simulink model "building_PHPP_v1"  (R2018b)
settings: Solver=ode23s  StartTime=-building.preruntime+8760*3600  StopTime=building.runtime+8760*3600  EnableMultiTasking=on
StartFcn:
  | tic
StopFcn:
  | toc
values from neighbouring files (symbols this model uses):
  A = 7*10*2    (= 140)    [theta_ground_v1.m]    (also in xlswrite1.m = num2cell(data))
  B = A/(0.5 * P)    (= 8.23529411765)    [theta_ground_v1.m]
  building = obj    [BUILDING.m]    (also in create_building_automatic.m = building.save(); ini_building_automatic.m = building.add_variant_hvac(building.variant_hvac, hvac); load_building_automatic.m = building.save())
  C = zeros(1,length(d)+1)    [CONSTRUCTION.m]    (also in DOOR.m = [0 0 0]; WALL.m = [0 0 0]; WINDOW.m = [0 0 0])
  cp = str2num(value)    [CONSTRUCTION.m]
  p = [timevec_weather weather(:,12)]    [BOUNDARY.m]    (also in WEATHER.m = 0; init_carnotUIBK.m = cell2mat(carnotUIBKpaths(i,2)))
  rho = str2num(value)    [CONSTRUCTION.m]    (also in theta_ground_v1.m = 2000)
undefined symbols (not defined in the file or in its folder): Dd, Dreifach, get_building, Qdot_C, Qdot_C_energy, Qdot_H, Qdot_H_energy, Qdot_I_electricity, Qdot_I_electricity_energy, Qdot_I_light, Qdot_I_light_energy, Qdot_I_person, Qdot_I_person_energy, Qdot_S, Qdot_S_energy, Qdot_T_ground, Qdot_T_ground_energy, Qdot_T_neighbour, Qdot_T_neighbour_energy, Qdot_T_opaque, Qdot_T_opaque_energy, Qdot_T_window, Qdot_T_window_energy, Qdot_V_infiltration, Qdot_V_infiltration_energy, Qdot_V_mech, Qdot_V_mech_energy, Qdot_V_window, Qdot_V_window_energy, Tc, Tr, Ts, Wärmeschutzglas, x_CO2, x_H2O, x_VOC
libraries: carnotUIBK x1874, carnot x5, simulink x3
(part 32 of 34)

== system building_PHPP_v1/BUILDING/ZONE_9/gain_4 ==
  AIB : Inport
  control : Inport  Port=2
  EMPTY : carnotUIBK/gain/EMPTY  SystemSampleTime=-1  VariantControl=(default)
  Equipment : carnotUIBK/gain/Equipment  SystemSampleTime=-1  VariantControl=V_z9_i4_m2
  Light : carnotUIBK/gain/Light  SystemSampleTime=-1  VariantControl=V_z9_i4_m1
  Moisture : carnotUIBK/gain/Moisture  SystemSampleTime=-1  VariantControl=V_z9_i4_m3
  People : carnotUIBK/gain/People  SystemSampleTime=-1  VariantControl=V_z9_i4_m0
  "[S]" : Outport

== system building_PHPP_v1/BUILDING/ZONE_9/gain_5 ==
  AIB : Inport
  control : Inport  Port=2
  EMPTY : carnotUIBK/gain/EMPTY  SystemSampleTime=-1  VariantControl=(default)
  Equipment : carnotUIBK/gain/Equipment  SystemSampleTime=-1  VariantControl=V_z9_i5_m2
  Light : carnotUIBK/gain/Light  SystemSampleTime=-1  VariantControl=V_z9_i5_m1
  Moisture : carnotUIBK/gain/Moisture  SystemSampleTime=-1  VariantControl=V_z9_i5_m3
  People : carnotUIBK/gain/People  SystemSampleTime=-1  VariantControl=V_z9_i5_m0
  "[S]" : Outport

== system building_PHPP_v1/BUILDING/ZONE_9/infiltration_1 ==
  AIB : Inport
  WDB : Inport  Port=2
  control : Inport  Port=3
  EMPTY : carnotUIBK/infiltration/EMPTY  VariantControl=(default)
  infiltration_constant : carnotUIBK/infiltration/infiltration_constant  VariantControl=V_z9_inf1_m0  volume=z.heated_volume  n50=z.n50  wind_e=0.07  co2=400
  infiltration_pressure : carnotUIBK/infiltration/infiltration_pressure  VariantControl=V_z9_inf1_m1  volume=z.heated_volume  n50=z.n50  wind_e=0.07  co2=400
  "[S]" : Outport

== system building_PHPP_v1/BUILDING/ZONE_9/infiltration_2 ==
  AIB : Inport
  WDB : Inport  Port=2
  control : Inport  Port=3
  EMPTY : carnotUIBK/infiltration/EMPTY  VariantControl=(default)
  infiltration_constant : carnotUIBK/infiltration/infiltration_constant  VariantControl=V_z9_inf2_m0  volume=z.heated_volume  n50=z.n50  wind_e=0.07  co2=400
  infiltration_pressure : carnotUIBK/infiltration/infiltration_pressure  VariantControl=V_z9_inf2_m1  volume=z.heated_volume  n50=z.n50  wind_e=0.07  co2=400
  "[S]" : Outport

== system building_PHPP_v1/BUILDING/ZONE_9/infiltration_3 ==
  AIB : Inport
  WDB : Inport  Port=2
  control : Inport  Port=3
  EMPTY : carnotUIBK/infiltration/EMPTY  VariantControl=(default)
  infiltration_constant : carnotUIBK/infiltration/infiltration_constant  VariantControl=V_z9_inf3_m0  volume=z.heated_volume  n50=z.n50  wind_e=0.07  co2=400
  infiltration_pressure : carnotUIBK/infiltration/infiltration_pressure  VariantControl=V_z9_inf3_m1  volume=z.heated_volume  n50=z.n50  wind_e=0.07  co2=400
  "[S]" : Outport

== system building_PHPP_v1/BUILDING/ZONE_9/infiltration_4 ==
  AIB : Inport
  WDB : Inport  Port=2
  control : Inport  Port=3
  EMPTY : carnotUIBK/infiltration/EMPTY  VariantControl=(default)
  infiltration_constant : carnotUIBK/infiltration/infiltration_constant  VariantControl=V_z9_inf4_m0  volume=z.heated_volume  n50=z.n50  wind_e=0.07  co2=400
  infiltration_pressure : carnotUIBK/infiltration/infiltration_pressure  VariantControl=V_z9_inf4_m1  volume=z.heated_volume  n50=z.n50  wind_e=0.07  co2=400
  "[S]" : Outport

== system building_PHPP_v1/BUILDING/ZONE_9/infiltration_5 ==
  AIB : Inport
  WDB : Inport  Port=2
  control : Inport  Port=3
  EMPTY : carnotUIBK/infiltration/EMPTY  VariantControl=(default)
  infiltration_constant : carnotUIBK/infiltration/infiltration_constant  VariantControl=V_z9_inf5_m0  volume=z.heated_volume  n50=z.n50  wind_e=0.07  co2=400
  infiltration_pressure : carnotUIBK/infiltration/infiltration_pressure  VariantControl=V_z9_inf5_m1  volume=z.heated_volume  n50=z.n50  wind_e=0.07  co2=400
  "[S]" : Outport

== system building_PHPP_v1/BUILDING/ZONE_9/room_node ==
  sum([S]) : Inport
  1-node : carnotUIBK/room_node/1-node  VariantControl=V_z9_m2  zoneairvolume=z.heated_volume  zoneheight=z.heated_volume/z.heated_area  zonestartTEMP=z.t_ini  zonestartWATER=z.phi_ini  zonestartCO2=z.CO2_ini  zonestartVOC=z.VOC_ini  zonestartP0=1e5/(293.15)*(273.15+z.t_ini)  timeconst=z.timeconstant  mcp=z.cp_spec*z.heated_area
  1-node_womass : carnotUIBK/room_node/1-node_womass  VariantControl=V_z9_m4  zoneairvolume=z.heated_volume  zoneheight=z.heated_volume/z.heated_area  zonestartTEMP=z.t_ini  zonestartWATER=z.phi_ini  zonestartCO2=z.CO2_ini  zonestartVOC=z.VOC_ini  zonestartP0=1e5/(293.15)*(273.15+z.t_ini)  timeconst=z.timeconstant  mcp=z.cp_spec*z.heated_area
  2-node : carnotUIBK/room_node/2-node  VariantControl=V_z9_m3  zoneairvolume=z.heated_volume  zoneheight=z.heated_volume/z.heated_area  zonestartTEMP=z.t_ini  zonestartWATER=z.phi_ini  zonestartCO2=z.CO2_ini  zonestartVOC=z.VOC_ini  zonestartP0=1e5/(293.15)*(273.15+z.t_ini)  timeconst=z.timeconstant
  2-node_ideal : carnotUIBK/room_node/2-node_ideal  VariantControl=V_z9_m1  zoneairvolume=z.heated_volume  zoneheight=z.heated_volume/z.heated_area  zonestartTEMP=z.t_ini  zonestartWATER=z.phi_ini  zonestartCO2=z.CO2_ini  zonestartVOC=z.VOC_ini  zonestartP0=1e5/(293.15)*(273.15+z.t_ini)  timeconst=z.timeconstant  temperature_timevalues=z.profile_timevalues  temperature_timeduration=z.profile_timeduration  temperature_Tc=z.profile_Tc  temperature_Tr=z.profile_Tc
  EMPTY : carnotUIBK/room_node/EMPTY  VariantControl=(default)  temperature_timevalues=z.profile_timevalues  temperature_timeduration=z.profile_timeduration  temperature_Tc=z.profile_Tc  temperature_Tr=z.profile_Tr  temperature_rH=z.profile_rH  temperature_CO2=z.profile_CO2  temperature_VOC=z.profile_VOC  temperature_p=z.profile_p
  BDB : Outport
  AIB : Outport  Port=2
  Qdot_sol : Outport  Port=3

== system building_PHPP_v1/BUILDING/ZONE_9/wall_1 ==
  WDB : Inport
  GDB : Inport  Port=2
  NDB : Inport  Port=3
  AIB : Inport  Port=4
  Qdot_in : Inport  Port=5
  Qdot_sol : Inport  Port=6
  EMPTY : carnotUIBK/wall_zone/EMPTY  VariantControl=(default)
  R-C model : carnotUIBK/wall_zone/R-C model  VariantControl=V_z9_w1_m1  t0=z.t_ini  d=fliplr(const.parameter.xmesh_beu)  cond=fliplr(const.parameter.lambda)  cwall=fliplr(const.parameter.cp)  rho=fliplr(const.parameter.rho)  reflectground=0.2  abs_emiss=[const.absorption_2 const.emission_2 const.emission_1]  tau=const.parameter.tau  dactive=const.parameter.d_active
      link override alpha_e/alpha_e_AMBIENT: VariantControl=V_z9_w1_hte0
      link override alpha_e/alpha_e_GROUND: VariantControl=V_z9_w1_hte1
      link override alpha_e/alpha_e_INTERNAL: VariantControl=V_z9_w1_hte2
      link override alpha_e/alpha_e_INTERNAL/alpha_i/alpha_i_down: VariantControl=V_z9_w1_hti2
      link override alpha_e/alpha_e_INTERNAL/alpha_i/alpha_i_horizontal: VariantControl=V_z9_w1_hti0
      link override alpha_e/alpha_e_INTERNAL/alpha_i/alpha_i_up: VariantControl=V_z9_w1_hti1
      link override alpha_e/alpha_e_NEIGHBOUR: VariantControl=V_z9_w1_hte3
      link override alpha_e/alpha_e_NEIGHBOUR/alpha_i/alpha_i_down: VariantControl=V_z9_w1_hti2
      link override alpha_e/alpha_e_NEIGHBOUR/alpha_i/alpha_i_horizontal: VariantControl=V_z9_w1_hti0
      link override alpha_e/alpha_e_NEIGHBOUR/alpha_i/alpha_i_up: VariantControl=V_z9_w1_hti1
      link override alpha_i/alpha_i_down: VariantControl=V_z9_w1_hti2
      link override alpha_i/alpha_i_horizontal: VariantControl=V_z9_w1_hti0
      link override alpha_i/alpha_i_up: VariantControl=V_z9_w1_hti1
  UA : carnotUIBK/wall_zone/UA  VariantControl=V_z9_w1_m0  U=const.parameter.U
      link override Rse/AMBIENT: VariantControl=V_z9_w1_hte0
      link override Rse/GROUND: VariantControl=V_z9_w1_hte1
      link override Rse/INTERNAL: VariantControl=V_z9_w1_hte2
      link override Rse/NEIGHBOUR: VariantControl=V_z9_w1_hte3
      link override Rsi/down: VariantControl=V_z9_w1_hti2
      link override Rsi/horizontal: VariantControl=V_z9_w1_hti0
      link override Rsi/up: VariantControl=V_z9_w1_hti1
  hygrothermal model : carnotUIBK/wall_zone/hygrothermal model  VariantControl=V_z9_w1_m2  t0=z.t_ini  reflectground=0.2  abs_emiss=[const.absorption_2 const.emission_2 const.emission_1]  xmesh=const.parameter.xmesh_hygro  X=const.parameter.X  d=const.parameter.d  lambda=const.parameter.lambda_hygro  rho=const.parameter.rho_hygro  cp=const.parameter.cp_hygro  mu=const.parameter.mu  ufs=const.parameter.ufs  FSF_u=const.parameter.FSF_u  FSF_phi=const.parameter.FSF_phi  FSF_dudphi=const.parameter.FSF_dudphi  FSF_k=const.parameter.FSF_k  K_kleff=const.parameter.K_kleff  K_u=const.parameter.K_u  K_kl=const.parameter.K_kl  FSF_length=const.parameter.FSF_length  K_length=const.parameter.K_length  T_ini=const.parameter.T_ini_hygro  Phi_ini=const.parameter.Phi_ini_hygro  T_source=const.parameter.T_source  Phi_source=const.parameter.Phi_source  Tdactive=const.parameter.T_dactive  Phidactive=const.parameter.Phi_dactive
      link override alpha_e/alpha_e_AMBIENT: VariantControl=V_z9_w1_hte0
      link override alpha_e/alpha_e_GROUND: VariantControl=V_z9_w1_hte1
      link override alpha_e/alpha_e_INTERNAL: VariantControl=V_z9_w1_hte2
      link override alpha_e/alpha_e_INTERNAL/alpha_i/alpha_i_down: VariantControl=V_z9_w1_hti2
      link override alpha_e/alpha_e_INTERNAL/alpha_i/alpha_i_horizontal: VariantControl=V_z9_w1_hti0
      link override alpha_e/alpha_e_INTERNAL/alpha_i/alpha_i_up: VariantControl=V_z9_w1_hti1
      link override alpha_e/alpha_e_NEIGHBOUR: VariantControl=V_z9_w1_hte3
      link override alpha_e/alpha_e_NEIGHBOUR/alpha_i/alpha_i_down: VariantControl=V_z9_w1_hti2
      link override alpha_e/alpha_e_NEIGHBOUR/alpha_i/alpha_i_horizontal: VariantControl=V_z9_w1_hti0
      link override alpha_e/alpha_e_NEIGHBOUR/alpha_i/alpha_i_up: VariantControl=V_z9_w1_hti1
      link override alpha_i/alpha_i_down: VariantControl=V_z9_w1_hti2
      link override alpha_i/alpha_i_horizontal: VariantControl=V_z9_w1_hti0
      link override alpha_i/alpha_i_up: VariantControl=V_z9_w1_hti1
  "[S]" : Outport
  theta_out : Outport  Port=2

== system building_PHPP_v1/BUILDING/ZONE_9/wall_2 ==
  WDB : Inport
  GDB : Inport  Port=2
  NDB : Inport  Port=3
  AIB : Inport  Port=4
  Qdot_in : Inport  Port=5
  Qdot_sol : Inport  Port=6
  EMPTY : carnotUIBK/wall_zone/EMPTY  VariantControl=(default)
  R-C model : carnotUIBK/wall_zone/R-C model  VariantControl=V_z9_w2_m1  t0=z.t_ini  d=fliplr(const.parameter.xmesh_beu)  cond=fliplr(const.parameter.lambda)  cwall=fliplr(const.parameter.cp)  rho=fliplr(const.parameter.rho)  reflectground=0.2  abs_emiss=[const.absorption_2 const.emission_2 const.emission_1]  tau=const.parameter.tau  dactive=const.parameter.d_active
      link override alpha_e/alpha_e_AMBIENT: VariantControl=V_z9_w2_hte0
      link override alpha_e/alpha_e_GROUND: VariantControl=V_z9_w2_hte1
      link override alpha_e/alpha_e_INTERNAL: VariantControl=V_z9_w2_hte2
      link override alpha_e/alpha_e_INTERNAL/alpha_i/alpha_i_down: VariantControl=V_z9_w2_hti2
      link override alpha_e/alpha_e_INTERNAL/alpha_i/alpha_i_horizontal: VariantControl=V_z9_w2_hti0
      link override alpha_e/alpha_e_INTERNAL/alpha_i/alpha_i_up: VariantControl=V_z9_w2_hti1
      link override alpha_e/alpha_e_NEIGHBOUR: VariantControl=V_z9_w2_hte3
      link override alpha_e/alpha_e_NEIGHBOUR/alpha_i/alpha_i_down: VariantControl=V_z9_w2_hti2
      link override alpha_e/alpha_e_NEIGHBOUR/alpha_i/alpha_i_horizontal: VariantControl=V_z9_w2_hti0
      link override alpha_e/alpha_e_NEIGHBOUR/alpha_i/alpha_i_up: VariantControl=V_z9_w2_hti1
      link override alpha_i/alpha_i_down: VariantControl=V_z9_w2_hti2
      link override alpha_i/alpha_i_horizontal: VariantControl=V_z9_w2_hti0
      link override alpha_i/alpha_i_up: VariantControl=V_z9_w2_hti1
  UA : carnotUIBK/wall_zone/UA  VariantControl=V_z9_w2_m0  U=const.parameter.U
      link override Rse/AMBIENT: VariantControl=V_z9_w2_hte0
      link override Rse/GROUND: VariantControl=V_z9_w2_hte1
      link override Rse/INTERNAL: VariantControl=V_z9_w2_hte2
      link override Rse/NEIGHBOUR: VariantControl=V_z9_w2_hte3
      link override Rsi/down: VariantControl=V_z9_w2_hti2
      link override Rsi/horizontal: VariantControl=V_z9_w2_hti0
      link override Rsi/up: VariantControl=V_z9_w2_hti1
  hygrothermal model : carnotUIBK/wall_zone/hygrothermal model  VariantControl=V_z9_w2_m2  t0=z.t_ini  reflectground=0.2  abs_emiss=[const.absorption_2 const.emission_2 const.emission_1]  xmesh=const.parameter.xmesh_hygro  X=const.parameter.X  d=const.parameter.d  lambda=const.parameter.lambda_hygro  rho=const.parameter.rho_hygro  cp=const.parameter.cp_hygro  mu=const.parameter.mu  ufs=const.parameter.ufs  FSF_u=const.parameter.FSF_u  FSF_phi=const.parameter.FSF_phi  FSF_dudphi=const.parameter.FSF_dudphi  FSF_k=const.parameter.FSF_k  K_kleff=const.parameter.K_kleff  K_u=const.parameter.K_u  K_kl=const.parameter.K_kl  FSF_length=const.parameter.FSF_length  K_length=const.parameter.K_length  T_ini=const.parameter.T_ini_hygro  Phi_ini=const.parameter.Phi_ini_hygro  T_source=const.parameter.T_source  Phi_source=const.parameter.Phi_source  Tdactive=const.parameter.T_dactive  Phidactive=const.parameter.Phi_dactive
      link override alpha_e/alpha_e_AMBIENT: VariantControl=V_z9_w2_hte0
      link override alpha_e/alpha_e_GROUND: VariantControl=V_z9_w2_hte1
      link override alpha_e/alpha_e_INTERNAL: VariantControl=V_z9_w2_hte2
      link override alpha_e/alpha_e_INTERNAL/alpha_i/alpha_i_down: VariantControl=V_z9_w2_hti2
      link override alpha_e/alpha_e_INTERNAL/alpha_i/alpha_i_horizontal: VariantControl=V_z9_w2_hti0
      link override alpha_e/alpha_e_INTERNAL/alpha_i/alpha_i_up: VariantControl=V_z9_w2_hti1
      link override alpha_e/alpha_e_NEIGHBOUR: VariantControl=V_z9_w2_hte3
      link override alpha_e/alpha_e_NEIGHBOUR/alpha_i/alpha_i_down: VariantControl=V_z9_w2_hti2
      link override alpha_e/alpha_e_NEIGHBOUR/alpha_i/alpha_i_horizontal: VariantControl=V_z9_w2_hti0
      link override alpha_e/alpha_e_NEIGHBOUR/alpha_i/alpha_i_up: VariantControl=V_z9_w2_hti1
      link override alpha_i/alpha_i_down: VariantControl=V_z9_w2_hti2
      link override alpha_i/alpha_i_horizontal: VariantControl=V_z9_w2_hti0
      link override alpha_i/alpha_i_up: VariantControl=V_z9_w2_hti1
  "[S]" : Outport
  theta_out : Outport  Port=2

== system building_PHPP_v1/BUILDING/ZONE_9/wall_3 ==
  WDB : Inport
  GDB : Inport  Port=2
  NDB : Inport  Port=3
  AIB : Inport  Port=4
  Qdot_in : Inport  Port=5
  Qdot_sol : Inport  Port=6
  EMPTY : carnotUIBK/wall_zone/EMPTY  VariantControl=(default)
  R-C model : carnotUIBK/wall_zone/R-C model  VariantControl=V_z9_w3_m1  t0=z.t_ini  d=fliplr(const.parameter.xmesh_beu)  cond=fliplr(const.parameter.lambda)  cwall=fliplr(const.parameter.cp)  rho=fliplr(const.parameter.rho)  reflectground=0.2  abs_emiss=[const.absorption_2 const.emission_2 const.emission_1]  tau=const.parameter.tau  dactive=const.parameter.d_active
      link override alpha_e/alpha_e_AMBIENT: VariantControl=V_z9_w3_hte0
      link override alpha_e/alpha_e_GROUND: VariantControl=V_z9_w3_hte1
      link override alpha_e/alpha_e_INTERNAL: VariantControl=V_z9_w3_hte2
      link override alpha_e/alpha_e_INTERNAL/alpha_i/alpha_i_down: VariantControl=V_z9_w3_hti2
      link override alpha_e/alpha_e_INTERNAL/alpha_i/alpha_i_horizontal: VariantControl=V_z9_w3_hti0
      link override alpha_e/alpha_e_INTERNAL/alpha_i/alpha_i_up: VariantControl=V_z9_w3_hti1
      link override alpha_e/alpha_e_NEIGHBOUR: VariantControl=V_z9_w3_hte3
      link override alpha_e/alpha_e_NEIGHBOUR/alpha_i/alpha_i_down: VariantControl=V_z9_w3_hti2
      link override alpha_e/alpha_e_NEIGHBOUR/alpha_i/alpha_i_horizontal: VariantControl=V_z9_w3_hti0
      link override alpha_e/alpha_e_NEIGHBOUR/alpha_i/alpha_i_up: VariantControl=V_z9_w3_hti1
      link override alpha_i/alpha_i_down: VariantControl=V_z9_w3_hti2
      link override alpha_i/alpha_i_horizontal: VariantControl=V_z9_w3_hti0
      link override alpha_i/alpha_i_up: VariantControl=V_z9_w3_hti1
  UA : carnotUIBK/wall_zone/UA  VariantControl=V_z9_w3_m0  U=const.parameter.U
      link override Rse/AMBIENT: VariantControl=V_z9_w3_hte0
      link override Rse/GROUND: VariantControl=V_z9_w3_hte1
      link override Rse/INTERNAL: VariantControl=V_z9_w3_hte2
      link override Rse/NEIGHBOUR: VariantControl=V_z9_w3_hte3
      link override Rsi/down: VariantControl=V_z9_w3_hti2
      link override Rsi/horizontal: VariantControl=V_z9_w3_hti0
      link override Rsi/up: VariantControl=V_z9_w3_hti1
  hygrothermal model : carnotUIBK/wall_zone/hygrothermal model  VariantControl=V_z9_w3_m2  t0=z.t_ini  reflectground=0.2  abs_emiss=[const.absorption_2 const.emission_2 const.emission_1]  xmesh=const.parameter.xmesh_hygro  X=const.parameter.X  d=const.parameter.d  lambda=const.parameter.lambda_hygro  rho=const.parameter.rho_hygro  cp=const.parameter.cp_hygro  mu=const.parameter.mu  ufs=const.parameter.ufs  FSF_u=const.parameter.FSF_u  FSF_phi=const.parameter.FSF_phi  FSF_dudphi=const.parameter.FSF_dudphi  FSF_k=const.parameter.FSF_k  K_kleff=const.parameter.K_kleff  K_u=const.parameter.K_u  K_kl=const.parameter.K_kl  FSF_length=const.parameter.FSF_length  K_length=const.parameter.K_length  T_ini=const.parameter.T_ini_hygro  Phi_ini=const.parameter.Phi_ini_hygro  T_source=const.parameter.T_source  Phi_source=const.parameter.Phi_source  Tdactive=const.parameter.T_dactive  Phidactive=const.parameter.Phi_dactive
      link override alpha_e/alpha_e_AMBIENT: VariantControl=V_z9_w3_hte0
      link override alpha_e/alpha_e_GROUND: VariantControl=V_z9_w3_hte1
      link override alpha_e/alpha_e_INTERNAL: VariantControl=V_z9_w3_hte2
      link override alpha_e/alpha_e_INTERNAL/alpha_i/alpha_i_down: VariantControl=V_z9_w3_hti2
      link override alpha_e/alpha_e_INTERNAL/alpha_i/alpha_i_horizontal: VariantControl=V_z9_w3_hti0
      link override alpha_e/alpha_e_INTERNAL/alpha_i/alpha_i_up: VariantControl=V_z9_w3_hti1
      link override alpha_e/alpha_e_NEIGHBOUR: VariantControl=V_z9_w3_hte3
      link override alpha_e/alpha_e_NEIGHBOUR/alpha_i/alpha_i_down: VariantControl=V_z9_w3_hti2
      link override alpha_e/alpha_e_NEIGHBOUR/alpha_i/alpha_i_horizontal: VariantControl=V_z9_w3_hti0
      link override alpha_e/alpha_e_NEIGHBOUR/alpha_i/alpha_i_up: VariantControl=V_z9_w3_hti1
      link override alpha_i/alpha_i_down: VariantControl=V_z9_w3_hti2
      link override alpha_i/alpha_i_horizontal: VariantControl=V_z9_w3_hti0
      link override alpha_i/alpha_i_up: VariantControl=V_z9_w3_hti1
  "[S]" : Outport
  theta_out : Outport  Port=2

== system building_PHPP_v1/BUILDING/ZONE_9/wall_4 ==
  WDB : Inport
  GDB : Inport  Port=2
  NDB : Inport  Port=3
  AIB : Inport  Port=4
  Qdot_in : Inport  Port=5
  Qdot_sol : Inport  Port=6
  EMPTY : carnotUIBK/wall_zone/EMPTY  VariantControl=(default)
  R-C model : carnotUIBK/wall_zone/R-C model  VariantControl=V_z9_w4_m1  t0=z.t_ini  d=fliplr(const.parameter.xmesh_beu)  cond=fliplr(const.parameter.lambda)  cwall=fliplr(const.parameter.cp)  rho=fliplr(const.parameter.rho)  reflectground=0.2  abs_emiss=[const.absorption_2 const.emission_2 const.emission_1]  tau=const.parameter.tau  dactive=const.parameter.d_active
      link override alpha_e/alpha_e_AMBIENT: VariantControl=V_z9_w4_hte0
      link override alpha_e/alpha_e_GROUND: VariantControl=V_z9_w4_hte1
      link override alpha_e/alpha_e_INTERNAL: VariantControl=V_z9_w4_hte2
      link override alpha_e/alpha_e_INTERNAL/alpha_i/alpha_i_down: VariantControl=V_z9_w4_hti2
      link override alpha_e/alpha_e_INTERNAL/alpha_i/alpha_i_horizontal: VariantControl=V_z9_w4_hti0
      link override alpha_e/alpha_e_INTERNAL/alpha_i/alpha_i_up: VariantControl=V_z9_w4_hti1
      link override alpha_e/alpha_e_NEIGHBOUR: VariantControl=V_z9_w4_hte3
      link override alpha_e/alpha_e_NEIGHBOUR/alpha_i/alpha_i_down: VariantControl=V_z9_w4_hti2
      link override alpha_e/alpha_e_NEIGHBOUR/alpha_i/alpha_i_horizontal: VariantControl=V_z9_w4_hti0
      link override alpha_e/alpha_e_NEIGHBOUR/alpha_i/alpha_i_up: VariantControl=V_z9_w4_hti1
      link override alpha_i/alpha_i_down: VariantControl=V_z9_w4_hti2
      link override alpha_i/alpha_i_horizontal: VariantControl=V_z9_w4_hti0
      link override alpha_i/alpha_i_up: VariantControl=V_z9_w4_hti1
  UA : carnotUIBK/wall_zone/UA  VariantControl=V_z9_w4_m0  U=const.parameter.U
      link override Rse/AMBIENT: VariantControl=V_z9_w4_hte0
      link override Rse/GROUND: VariantControl=V_z9_w4_hte1
      link override Rse/INTERNAL: VariantControl=V_z9_w4_hte2
      link override Rse/NEIGHBOUR: VariantControl=V_z9_w4_hte3
      link override Rsi/down: VariantControl=V_z9_w4_hti2
      link override Rsi/horizontal: VariantControl=V_z9_w4_hti0
      link override Rsi/up: VariantControl=V_z9_w4_hti1
  hygrothermal model : carnotUIBK/wall_zone/hygrothermal model  VariantControl=V_z9_w4_m2  t0=z.t_ini  reflectground=0.2  abs_emiss=[const.absorption_2 const.emission_2 const.emission_1]  xmesh=const.parameter.xmesh_hygro  X=const.parameter.X  d=const.parameter.d  lambda=const.parameter.lambda_hygro  rho=const.parameter.rho_hygro  cp=const.parameter.cp_hygro  mu=const.parameter.mu  ufs=const.parameter.ufs  FSF_u=const.parameter.FSF_u  FSF_phi=const.parameter.FSF_phi  FSF_dudphi=const.parameter.FSF_dudphi  FSF_k=const.parameter.FSF_k  K_kleff=const.parameter.K_kleff  K_u=const.parameter.K_u  K_kl=const.parameter.K_kl  FSF_length=const.parameter.FSF_length  K_length=const.parameter.K_length  T_ini=const.parameter.T_ini_hygro  Phi_ini=const.parameter.Phi_ini_hygro  T_source=const.parameter.T_source  Phi_source=const.parameter.Phi_source  Tdactive=const.parameter.T_dactive  Phidactive=const.parameter.Phi_dactive
      link override alpha_e/alpha_e_AMBIENT: VariantControl=V_z9_w4_hte0
      link override alpha_e/alpha_e_GROUND: VariantControl=V_z9_w4_hte1
      link override alpha_e/alpha_e_INTERNAL: VariantControl=V_z9_w4_hte2
      link override alpha_e/alpha_e_INTERNAL/alpha_i/alpha_i_down: VariantControl=V_z9_w4_hti2
      link override alpha_e/alpha_e_INTERNAL/alpha_i/alpha_i_horizontal: VariantControl=V_z9_w4_hti0
      link override alpha_e/alpha_e_INTERNAL/alpha_i/alpha_i_up: VariantControl=V_z9_w4_hti1
      link override alpha_e/alpha_e_NEIGHBOUR: VariantControl=V_z9_w4_hte3
      link override alpha_e/alpha_e_NEIGHBOUR/alpha_i/alpha_i_down: VariantControl=V_z9_w4_hti2
      link override alpha_e/alpha_e_NEIGHBOUR/alpha_i/alpha_i_horizontal: VariantControl=V_z9_w4_hti0
      link override alpha_e/alpha_e_NEIGHBOUR/alpha_i/alpha_i_up: VariantControl=V_z9_w4_hti1
      link override alpha_i/alpha_i_down: VariantControl=V_z9_w4_hti2
      link override alpha_i/alpha_i_horizontal: VariantControl=V_z9_w4_hti0
      link override alpha_i/alpha_i_up: VariantControl=V_z9_w4_hti1
  "[S]" : Outport
  theta_out : Outport  Port=2

== system building_PHPP_v1/BUILDING/ZONE_9/wall_5 ==
  WDB : Inport
  GDB : Inport  Port=2
  NDB : Inport  Port=3
  AIB : Inport  Port=4
  Qdot_in : Inport  Port=5
  Qdot_sol : Inport  Port=6
  EMPTY : carnotUIBK/wall_zone/EMPTY  VariantControl=(default)
  R-C model : carnotUIBK/wall_zone/R-C model  VariantControl=V_z9_w5_m1  t0=z.t_ini  d=fliplr(const.parameter.xmesh_beu)  cond=fliplr(const.parameter.lambda)  cwall=fliplr(const.parameter.cp)  rho=fliplr(const.parameter.rho)  reflectground=0.2  abs_emiss=[const.absorption_2 const.emission_2 const.emission_1]  tau=const.parameter.tau  dactive=const.parameter.d_active
      link override alpha_e/alpha_e_AMBIENT: VariantControl=V_z9_w5_hte0
      link override alpha_e/alpha_e_GROUND: VariantControl=V_z9_w5_hte1
      link override alpha_e/alpha_e_INTERNAL: VariantControl=V_z9_w5_hte2
      link override alpha_e/alpha_e_INTERNAL/alpha_i/alpha_i_down: VariantControl=V_z9_w5_hti2
      link override alpha_e/alpha_e_INTERNAL/alpha_i/alpha_i_horizontal: VariantControl=V_z9_w5_hti0
      link override alpha_e/alpha_e_INTERNAL/alpha_i/alpha_i_up: VariantControl=V_z9_w5_hti1
      link override alpha_e/alpha_e_NEIGHBOUR: VariantControl=V_z9_w5_hte3
      link override alpha_e/alpha_e_NEIGHBOUR/alpha_i/alpha_i_down: VariantControl=V_z9_w5_hti2
      link override alpha_e/alpha_e_NEIGHBOUR/alpha_i/alpha_i_horizontal: VariantControl=V_z9_w5_hti0
      link override alpha_e/alpha_e_NEIGHBOUR/alpha_i/alpha_i_up: VariantControl=V_z9_w5_hti1
      link override alpha_i/alpha_i_down: VariantControl=V_z9_w5_hti2
      link override alpha_i/alpha_i_horizontal: VariantControl=V_z9_w5_hti0
      link override alpha_i/alpha_i_up: VariantControl=V_z9_w5_hti1
  UA : carnotUIBK/wall_zone/UA  VariantControl=V_z9_w5_m0  U=const.parameter.U
      link override Rse/AMBIENT: VariantControl=V_z9_w5_hte0
      link override Rse/GROUND: VariantControl=V_z9_w5_hte1
      link override Rse/INTERNAL: VariantControl=V_z9_w5_hte2
      link override Rse/NEIGHBOUR: VariantControl=V_z9_w5_hte3
      link override Rsi/down: VariantControl=V_z9_w5_hti2
      link override Rsi/horizontal: VariantControl=V_z9_w5_hti0
      link override Rsi/up: VariantControl=V_z9_w5_hti1
  hygrothermal model : carnotUIBK/wall_zone/hygrothermal model  VariantControl=V_z9_w5_m2  t0=z.t_ini  reflectground=0.2  abs_emiss=[const.absorption_2 const.emission_2 const.emission_1]  xmesh=const.parameter.xmesh_hygro  X=const.parameter.X  d=const.parameter.d  lambda=const.parameter.lambda_hygro  rho=const.parameter.rho_hygro  cp=const.parameter.cp_hygro  mu=const.parameter.mu  ufs=const.parameter.ufs  FSF_u=const.parameter.FSF_u  FSF_phi=const.parameter.FSF_phi  FSF_dudphi=const.parameter.FSF_dudphi  FSF_k=const.parameter.FSF_k  K_kleff=const.parameter.K_kleff  K_u=const.parameter.K_u  K_kl=const.parameter.K_kl  FSF_length=const.parameter.FSF_length  K_length=const.parameter.K_length  T_ini=const.parameter.T_ini_hygro  Phi_ini=const.parameter.Phi_ini_hygro  T_source=const.parameter.T_source  Phi_source=const.parameter.Phi_source  Tdactive=const.parameter.T_dactive  Phidactive=const.parameter.Phi_dactive
      link override alpha_e/alpha_e_AMBIENT: VariantControl=V_z9_w5_hte0
      link override alpha_e/alpha_e_GROUND: VariantControl=V_z9_w5_hte1
      link override alpha_e/alpha_e_INTERNAL: VariantControl=V_z9_w5_hte2
      link override alpha_e/alpha_e_INTERNAL/alpha_i/alpha_i_down: VariantControl=V_z9_w5_hti2
      link override alpha_e/alpha_e_INTERNAL/alpha_i/alpha_i_horizontal: VariantControl=V_z9_w5_hti0
      link override alpha_e/alpha_e_INTERNAL/alpha_i/alpha_i_up: VariantControl=V_z9_w5_hti1
      link override alpha_e/alpha_e_NEIGHBOUR: VariantControl=V_z9_w5_hte3
      link override alpha_e/alpha_e_NEIGHBOUR/alpha_i/alpha_i_down: VariantControl=V_z9_w5_hti2
      link override alpha_e/alpha_e_NEIGHBOUR/alpha_i/alpha_i_horizontal: VariantControl=V_z9_w5_hti0
      link override alpha_e/alpha_e_NEIGHBOUR/alpha_i/alpha_i_up: VariantControl=V_z9_w5_hti1
      link override alpha_i/alpha_i_down: VariantControl=V_z9_w5_hti2
      link override alpha_i/alpha_i_horizontal: VariantControl=V_z9_w5_hti0
      link override alpha_i/alpha_i_up: VariantControl=V_z9_w5_hti1
  "[S]" : Outport
  theta_out : Outport  Port=2

== system building_PHPP_v1/BUILDING/ZONE_9/wall_6 ==
  WDB : Inport
  GDB : Inport  Port=2
  NDB : Inport  Port=3
  AIB : Inport  Port=4
  Qdot_in : Inport  Port=5
  Qdot_sol : Inport  Port=6
  EMPTY : carnotUIBK/wall_zone/EMPTY  VariantControl=(default)
  R-C model : carnotUIBK/wall_zone/R-C model  VariantControl=V_z9_w6_m1  t0=z.t_ini  d=fliplr(const.parameter.xmesh_beu)  cond=fliplr(const.parameter.lambda)  cwall=fliplr(const.parameter.cp)  rho=fliplr(const.parameter.rho)  reflectground=0.2  abs_emiss=[const.absorption_2 const.emission_2 const.emission_1]  tau=const.parameter.tau  dactive=const.parameter.d_active
      link override alpha_e/alpha_e_AMBIENT: VariantControl=V_z9_w6_hte0
      link override alpha_e/alpha_e_GROUND: VariantControl=V_z9_w6_hte1
      link override alpha_e/alpha_e_INTERNAL: VariantControl=V_z9_w6_hte2
      link override alpha_e/alpha_e_INTERNAL/alpha_i/alpha_i_down: VariantControl=V_z9_w6_hti2
      link override alpha_e/alpha_e_INTERNAL/alpha_i/alpha_i_horizontal: VariantControl=V_z9_w6_hti0
      link override alpha_e/alpha_e_INTERNAL/alpha_i/alpha_i_up: VariantControl=V_z9_w6_hti1
      link override alpha_e/alpha_e_NEIGHBOUR: VariantControl=V_z9_w6_hte3
      link override alpha_e/alpha_e_NEIGHBOUR/alpha_i/alpha_i_down: VariantControl=V_z9_w6_hti2
      link override alpha_e/alpha_e_NEIGHBOUR/alpha_i/alpha_i_horizontal: VariantControl=V_z9_w6_hti0
      link override alpha_e/alpha_e_NEIGHBOUR/alpha_i/alpha_i_up: VariantControl=V_z9_w6_hti1
      link override alpha_i/alpha_i_down: VariantControl=V_z9_w6_hti2
      link override alpha_i/alpha_i_horizontal: VariantControl=V_z9_w6_hti0
      link override alpha_i/alpha_i_up: VariantControl=V_z9_w6_hti1
  UA : carnotUIBK/wall_zone/UA  VariantControl=V_z9_w6_m0  U=const.parameter.U
      link override Rse/AMBIENT: VariantControl=V_z9_w6_hte0
      link override Rse/GROUND: VariantControl=V_z9_w6_hte1
      link override Rse/INTERNAL: VariantControl=V_z9_w6_hte2
      link override Rse/NEIGHBOUR: VariantControl=V_z9_w6_hte3
      link override Rsi/down: VariantControl=V_z9_w6_hti2
      link override Rsi/horizontal: VariantControl=V_z9_w6_hti0
      link override Rsi/up: VariantControl=V_z9_w6_hti1
  hygrothermal model : carnotUIBK/wall_zone/hygrothermal model  VariantControl=V_z9_w6_m2  t0=z.t_ini  reflectground=0.2  abs_emiss=[const.absorption_2 const.emission_2 const.emission_1]  xmesh=const.parameter.xmesh_hygro  X=const.parameter.X  d=const.parameter.d  lambda=const.parameter.lambda_hygro  rho=const.parameter.rho_hygro  cp=const.parameter.cp_hygro  mu=const.parameter.mu  ufs=const.parameter.ufs  FSF_u=const.parameter.FSF_u  FSF_phi=const.parameter.FSF_phi  FSF_dudphi=const.parameter.FSF_dudphi  FSF_k=const.parameter.FSF_k  K_kleff=const.parameter.K_kleff  K_u=const.parameter.K_u  K_kl=const.parameter.K_kl  FSF_length=const.parameter.FSF_length  K_length=const.parameter.K_length  T_ini=const.parameter.T_ini_hygro  Phi_ini=const.parameter.Phi_ini_hygro  T_source=const.parameter.T_source  Phi_source=const.parameter.Phi_source  Tdactive=const.parameter.T_dactive  Phidactive=const.parameter.Phi_dactive
      link override alpha_e/alpha_e_AMBIENT: VariantControl=V_z9_w6_hte0
      link override alpha_e/alpha_e_GROUND: VariantControl=V_z9_w6_hte1
      link override alpha_e/alpha_e_INTERNAL: VariantControl=V_z9_w6_hte2
      link override alpha_e/alpha_e_INTERNAL/alpha_i/alpha_i_down: VariantControl=V_z9_w6_hti2
      link override alpha_e/alpha_e_INTERNAL/alpha_i/alpha_i_horizontal: VariantControl=V_z9_w6_hti0
      link override alpha_e/alpha_e_INTERNAL/alpha_i/alpha_i_up: VariantControl=V_z9_w6_hti1
      link override alpha_e/alpha_e_NEIGHBOUR: VariantControl=V_z9_w6_hte3
      link override alpha_e/alpha_e_NEIGHBOUR/alpha_i/alpha_i_down: VariantControl=V_z9_w6_hti2
      link override alpha_e/alpha_e_NEIGHBOUR/alpha_i/alpha_i_horizontal: VariantControl=V_z9_w6_hti0
      link override alpha_e/alpha_e_NEIGHBOUR/alpha_i/alpha_i_up: VariantControl=V_z9_w6_hti1
      link override alpha_i/alpha_i_down: VariantControl=V_z9_w6_hti2
      link override alpha_i/alpha_i_horizontal: VariantControl=V_z9_w6_hti0
      link override alpha_i/alpha_i_up: VariantControl=V_z9_w6_hti1
  "[S]" : Outport
  theta_out : Outport  Port=2

== system building_PHPP_v1/BUILDING/ZONE_9/window_1 ==
  note: FORGET THIS STUPID MODEL!!!!
  WDB : Inport
  AIB : Inport  Port=2
  control : Inport  Port=3
  EMTPY : carnotUIBK/window/EMTPY  VariantControl=(default)
  window_CARNOT : carnotUIBK/window/window_CARNOT  VariantControl=V_z9_wi1_m1  wallsize=[window_heigth window_width]  frame=r_frame  pos=pos  t0=z.t_ini  d=const.parameter.d_w  cond=const.parameter.lambda_w  cwall=const.parameter.c_w  rho=const.parameter.rho_w  misc=[0.20 const.absorption_2 const.emission_2 const.emission_1]  gvalue=const.parameter.g_w  dactive=[0.01 0.05]
  window_TF : carnotUIBK/window/window_TF  VariantControl=V_z9_wi1_m0  windowsize=[window_heigth window_width]  numpanes=const.parameter.n_pane  frame=r_frame  pos=pos  d=const.parameter.d_w  rho=const.parameter.rho_w  cp=const.parameter.c_w  t0=z.t_ini  misc=[0.20 const.absorption_2 const.emission_2 const.emission_1]  gvalue=const.parameter.g_w  tauzero=const.parameter.tau_g_w  Ug=Uvalue  shad_type=No shading  type_glazing=Dreifach-Wärmeschutzglas  tau_shad=0.304  bli_a=0.08  bli_b=0.0126  bli_c=0.009  bli_d=0.062  bli_alpha=45  bli_refl=0.441
  window_TF_shading : carnotUIBK/window/window_TF_shading  VariantControl=V_z9_wi1_m2  windowsize=[window_heigth window_width]  numpanes=const.parameter.n_pane  frame=r_frame  pos=pos  d=const.parameter.d_w  rho=const.parameter.rho_w  cp=const.parameter.c_w  t0=z.t_ini  misc=[0.20 const.absorption_2 const.emission_2 const.emission_1]  gvalue=const.parameter.g_w  tauzero=const.parameter.tau_g_w  Ug=Uvalue  shad_type=Exterior Screen  type_glazing=Dreifach-Wärmeschutzglas  tau_shad=const.parameter.solar_transmittance  bli_a=const.parameter.venetianblind_a  bli_b=const.parameter.venetianblind_b  bli_c=const.parameter.venetianblind_c  bli_d=const.parameter.venetianblind_d  bli_alpha=const.parameter.venetianblind_angle  bli_refl=const.parameter.venetianblind_reflect
  "[S]" : Outport

== system building_PHPP_v1/BUILDING/ZONE_9/window_2 ==
  note: FORGET THIS STUPID MODEL!!!!
  WDB : Inport
  AIB : Inport  Port=2
  control : Inport  Port=3
  EMTPY : carnotUIBK/window/EMTPY  VariantControl=(default)
  window_CARNOT : carnotUIBK/window/window_CARNOT  VariantControl=V_z9_wi2_m1  wallsize=[window_heigth window_width]  frame=r_frame  pos=pos  t0=z.t_ini  d=const.parameter.d_w  cond=const.parameter.lambda_w  cwall=const.parameter.c_w  rho=const.parameter.rho_w  misc=[0.20 const.absorption_2 const.emission_2 const.emission_1]  gvalue=const.parameter.g_w  dactive=[0.01 0.05]
  window_TF : carnotUIBK/window/window_TF  VariantControl=V_z9_wi2_m0  windowsize=[window_heigth window_width]  numpanes=const.parameter.n_pane  frame=r_frame  pos=pos  d=const.parameter.d_w  rho=const.parameter.rho_w  cp=const.parameter.c_w  t0=z.t_ini  misc=[0.20 const.absorption_2 const.emission_2 const.emission_1]  gvalue=const.parameter.g_w  tauzero=const.parameter.tau_g_w  Ug=Uvalue  shad_type=No shading  type_glazing=Dreifach-Wärmeschutzglas  tau_shad=0.304  bli_a=0.08  bli_b=0.0126  bli_c=0.009  bli_d=0.062  bli_alpha=45  bli_refl=0.441
  window_TF_shading : carnotUIBK/window/window_TF_shading  VariantControl=V_z9_wi2_m2  windowsize=[window_heigth window_width]  numpanes=const.parameter.n_pane  frame=r_frame  pos=pos  d=const.parameter.d_w  rho=const.parameter.rho_w  cp=const.parameter.c_w  t0=z.t_ini  misc=[0.20 const.absorption_2 const.emission_2 const.emission_1]  gvalue=const.parameter.g_w  tauzero=const.parameter.tau_g_w  Ug=Uvalue  shad_type=Exterior Screen  type_glazing=Dreifach-Wärmeschutzglas  tau_shad=const.parameter.solar_transmittance  bli_a=const.parameter.venetianblind_a  bli_b=const.parameter.venetianblind_b  bli_c=const.parameter.venetianblind_c  bli_d=const.parameter.venetianblind_d  bli_alpha=const.parameter.venetianblind_angle  bli_refl=const.parameter.venetianblind_reflect
  "[S]" : Outport

== system building_PHPP_v1/BUILDING/ZONE_9/window_3 ==
  note: FORGET THIS STUPID MODEL!!!!
  WDB : Inport
  AIB : Inport  Port=2
  control : Inport  Port=3
  EMTPY : carnotUIBK/window/EMTPY  VariantControl=(default)
  window_CARNOT : carnotUIBK/window/window_CARNOT  VariantControl=V_z9_wi3_m1  wallsize=[window_heigth window_width]  frame=r_frame  pos=pos  t0=z.t_ini  d=const.parameter.d_w  cond=const.parameter.lambda_w  cwall=const.parameter.c_w  rho=const.parameter.rho_w  misc=[0.20 const.absorption_2 const.emission_2 const.emission_1]  gvalue=const.parameter.g_w  dactive=[0.01 0.05]
  window_TF : carnotUIBK/window/window_TF  VariantControl=V_z9_wi3_m0  windowsize=[window_heigth window_width]  numpanes=const.parameter.n_pane  frame=r_frame  pos=pos  d=const.parameter.d_w  rho=const.parameter.rho_w  cp=const.parameter.c_w  t0=z.t_ini  misc=[0.20 const.absorption_2 const.emission_2 const.emission_1]  gvalue=const.parameter.g_w  tauzero=const.parameter.tau_g_w  Ug=Uvalue  shad_type=No shading  type_glazing=Dreifach-Wärmeschutzglas  tau_shad=0.304  bli_a=0.08  bli_b=0.0126  bli_c=0.009  bli_d=0.062  bli_alpha=45  bli_refl=0.441
  window_TF_shading : carnotUIBK/window/window_TF_shading  VariantControl=V_z9_wi3_m2  windowsize=[window_heigth window_width]  numpanes=const.parameter.n_pane  frame=r_frame  pos=pos  d=const.parameter.d_w  rho=const.parameter.rho_w  cp=const.parameter.c_w  t0=z.t_ini  misc=[0.20 const.absorption_2 const.emission_2 const.emission_1]  gvalue=const.parameter.g_w  tauzero=const.parameter.tau_g_w  Ug=Uvalue  shad_type=Exterior Screen  type_glazing=Dreifach-Wärmeschutzglas  tau_shad=const.parameter.solar_transmittance  bli_a=const.parameter.venetianblind_a  bli_b=const.parameter.venetianblind_b  bli_c=const.parameter.venetianblind_c  bli_d=const.parameter.venetianblind_d  bli_alpha=const.parameter.venetianblind_angle  bli_refl=const.parameter.venetianblind_reflect
  "[S]" : Outport

== system building_PHPP_v1/BUILDING/ZONE_9/window_4 ==
  note: FORGET THIS STUPID MODEL!!!!
  WDB : Inport
  AIB : Inport  Port=2
  control : Inport  Port=3
  EMTPY : carnotUIBK/window/EMTPY  VariantControl=(default)
  window_CARNOT : carnotUIBK/window/window_CARNOT  VariantControl=V_z9_wi4_m1  wallsize=[window_heigth window_width]  frame=r_frame  pos=pos  t0=z.t_ini  d=const.parameter.d_w  cond=const.parameter.lambda_w  cwall=const.parameter.c_w  rho=const.parameter.rho_w  misc=[0.20 const.absorption_2 const.emission_2 const.emission_1]  gvalue=const.parameter.g_w  dactive=[0.01 0.05]
  window_TF : carnotUIBK/window/window_TF  VariantControl=V_z9_wi4_m0  windowsize=[window_heigth window_width]  numpanes=const.parameter.n_pane  frame=r_frame  pos=pos  d=const.parameter.d_w  rho=const.parameter.rho_w  cp=const.parameter.c_w  t0=z.t_ini  misc=[0.20 const.absorption_2 const.emission_2 const.emission_1]  gvalue=const.parameter.g_w  tauzero=const.parameter.tau_g_w  Ug=Uvalue  shad_type=No shading  type_glazing=Dreifach-Wärmeschutzglas  tau_shad=0.304  bli_a=0.08  bli_b=0.0126  bli_c=0.009  bli_d=0.062  bli_alpha=45  bli_refl=0.441
  window_TF_shading : carnotUIBK/window/window_TF_shading  VariantControl=V_z9_wi4_m2  windowsize=[window_heigth window_width]  numpanes=const.parameter.n_pane  frame=r_frame  pos=pos  d=const.parameter.d_w  rho=const.parameter.rho_w  cp=const.parameter.c_w  t0=z.t_ini  misc=[0.20 const.absorption_2 const.emission_2 const.emission_1]  gvalue=const.parameter.g_w  tauzero=const.parameter.tau_g_w  Ug=Uvalue  shad_type=Exterior Screen  type_glazing=Dreifach-Wärmeschutzglas  tau_shad=const.parameter.solar_transmittance  bli_a=const.parameter.venetianblind_a  bli_b=const.parameter.venetianblind_b  bli_c=const.parameter.venetianblind_c  bli_d=const.parameter.venetianblind_d  bli_alpha=const.parameter.venetianblind_angle  bli_refl=const.parameter.venetianblind_reflect
  "[S]" : Outport

== system building_PHPP_v1/BUILDING/ZONE_9/window_5 ==
  note: FORGET THIS STUPID MODEL!!!!
  WDB : Inport
  AIB : Inport  Port=2
  control : Inport  Port=3
  EMTPY : carnotUIBK/window/EMTPY  VariantControl=(default)
  window_CARNOT : carnotUIBK/window/window_CARNOT  VariantControl=V_z9_wi5_m1  wallsize=[window_heigth window_width]  frame=r_frame  pos=pos  t0=z.t_ini  d=const.parameter.d_w  cond=const.parameter.lambda_w  cwall=const.parameter.c_w  rho=const.parameter.rho_w  misc=[0.20 const.absorption_2 const.emission_2 const.emission_1]  gvalue=const.parameter.g_w  dactive=[0.01 0.05]
  window_TF : carnotUIBK/window/window_TF  VariantControl=V_z9_wi5_m0  windowsize=[window_heigth window_width]  numpanes=const.parameter.n_pane  frame=r_frame  pos=pos  d=const.parameter.d_w  rho=const.parameter.rho_w  cp=const.parameter.c_w  t0=z.t_ini  misc=[0.20 const.absorption_2 const.emission_2 const.emission_1]  gvalue=const.parameter.g_w  tauzero=const.parameter.tau_g_w  Ug=Uvalue  shad_type=No shading  type_glazing=Dreifach-Wärmeschutzglas  tau_shad=0.304  bli_a=0.08  bli_b=0.0126  bli_c=0.009  bli_d=0.062  bli_alpha=45  bli_refl=0.441
  window_TF_shading : carnotUIBK/window/window_TF_shading  VariantControl=V_z9_wi5_m2  windowsize=[window_heigth window_width]  numpanes=const.parameter.n_pane  frame=r_frame  pos=pos  d=const.parameter.d_w  rho=const.parameter.rho_w  cp=const.parameter.c_w  t0=z.t_ini  misc=[0.20 const.absorption_2 const.emission_2 const.emission_1]  gvalue=const.parameter.g_w  tauzero=const.parameter.tau_g_w  Ug=Uvalue  shad_type=Exterior Screen  type_glazing=Dreifach-Wärmeschutzglas  tau_shad=const.parameter.solar_transmittance  bli_a=const.parameter.venetianblind_a  bli_b=const.parameter.venetianblind_b  bli_c=const.parameter.venetianblind_c  bli_d=const.parameter.venetianblind_d  bli_alpha=const.parameter.venetianblind_angle  bli_refl=const.parameter.venetianblind_reflect
  "[S]" : Outport

== system building_PHPP_v1/DATALOGGER/logger_BDB/z1 ==
  BDB : Inport
  Bus Assignment : BusAssignment  AssignedSignals=Qdot_T_opaque_energy,Qdot_T_ground_energy,Qdot_T_neighbour_energy,Qdot_T_window_energy,Qdot_V_mech_energy,Qdot_V_window_energy,Qdot_V_infiltration_energy,Qdot_S_energy,Qdot_I_person_energy,Qdot_I_light_energy,Qdot_I_electricity_energy,Qdot_H_energy,Qdot_C_energy
  Bus Creator1 : BusCreator  Inputs=13
  Bus Selector1 : BusSelector  OutputSignals=z1.Qdot_T_opaque,z1.Qdot_T_ground,z1.Qdot_T_neighbour,z1.Qdot_T_window,z1.Qdot_V_mech,z1.Qdot_V_window,z1.Qdot_V_infiltration,z1.Qdot_S,z1.Qdot_I_person,z1.Qdot_I_light,z1.Qdot_I_electricity,z1.Qdot_H,z1.Qdot_C
  Constant{,1..12} (13 alike) : Constant  Value=0
  Subsystem : Subsystem
  Subsystem1 : Subsystem
  Subsystem10 : Subsystem
  Subsystem11 : Subsystem
  Subsystem12 : Subsystem
  Subsystem2 : Subsystem
  Subsystem3 : Subsystem
  Subsystem4 : Subsystem
  Subsystem5 : Subsystem
  Subsystem6 : Subsystem
  Subsystem7 : Subsystem
  Subsystem8 : Subsystem
  Subsystem9 : Subsystem
  BDBenergy : Outport
  wires:
  Constant12/1 -> Bus Creator1/13  "Qdot_C_energy"
  Constant2/1 -> Bus Creator1/3  "Qdot_T_neighbour_energy"
  Constant4/1 -> Bus Creator1/5  "Qdot_V_mech_energy"
  Constant9/1 -> Bus Creator1/10  "Qdot_I_light_energy"
  Constant1/1 -> Bus Creator1/2  "Qdot_T_ground_energy"
  Constant3/1 -> Bus Creator1/4  "Qdot_T_window_energy"
  Constant11/1 -> Bus Creator1/12  "Qdot_H_energy"
  Constant10/1 -> Bus Creator1/11  "Qdot_I_electricity_energy"
  Constant/1 -> Bus Creator1/1  "Qdot_T_opaque_energy"
  Constant8/1 -> Bus Creator1/8  "Qdot_S_energy"
  Constant7/1 -> Bus Creator1/9  "Qdot_I_person_energy"
  Constant6/1 -> Bus Creator1/7  "Qdot_V_infiltration_energy"
  BDB/1 -> Bus Selector1/1
  Constant5/1 -> Bus Creator1/6  "Qdot_V_window_energy"
  Bus Selector1/1 -> Subsystem/1(In1)  "<Qdot_T_opaque>"
  Bus Selector1/4 -> Subsystem3/1(In1)  "<Qdot_T_window>"
  Bus Selector1/3 -> Subsystem2/1(In1)  "<Qdot_T_neighbour>"
  Bus Selector1/2 -> Subsystem1/1(In1)  "<Qdot_T_ground>"
  Bus Selector1/9 -> Subsystem8/1(In1)  "<Qdot_I_person>"
  Bus Selector1/10 -> Subsystem9/1(In1)  "<Qdot_I_light>"
  Bus Selector1/11 -> Subsystem10/1(In1)  "<Qdot_I_electricity>"
  Bus Selector1/12 -> Subsystem11/1(In1)  "<Qdot_H>"
  Bus Selector1/13 -> Subsystem12/1(In1)  "<Qdot_C>"
  Bus Selector1/8 -> Subsystem7/1(In1)  "<Qdot_S>"
  Bus Selector1/7 -> Subsystem6/1(In1)  "<Qdot_V_infiltration>"
  Bus Selector1/6 -> Subsystem5/1(In1)  "<Qdot_V_window>"
  Bus Selector1/5 -> Subsystem4/1(In1)  "<Qdot_V_mech>"
  Bus Assignment/1 -> BDBenergy/1
  Bus Creator1/1 -> Bus Assignment/1
  Subsystem/1(Out1) -> Bus Assignment/2
  Subsystem12/1(Out1) -> Bus Assignment/14
  Subsystem11/1(Out1) -> Bus Assignment/13
  Subsystem10/1(Out1) -> Bus Assignment/12
  Subsystem9/1(Out1) -> Bus Assignment/11
  Subsystem8/1(Out1) -> Bus Assignment/10
  Subsystem7/1(Out1) -> Bus Assignment/9
  Subsystem6/1(Out1) -> Bus Assignment/8
  Subsystem5/1(Out1) -> Bus Assignment/7
  Subsystem4/1(Out1) -> Bus Assignment/6
  Subsystem3/1(Out1) -> Bus Assignment/5
  Subsystem2/1(Out1) -> Bus Assignment/4
  Subsystem1/1(Out1) -> Bus Assignment/3

== system building_PHPP_v1/DATALOGGER/logger_BDB/z10 ==
  BDB : Inport
  Bus Assignment : BusAssignment  AssignedSignals=Qdot_T_opaque_energy,Qdot_T_ground_energy,Qdot_T_neighbour_energy,Qdot_T_window_energy,Qdot_V_mech_energy,Qdot_V_window_energy,Qdot_V_infiltration_energy,Qdot_S_energy,Qdot_I_person_energy,Qdot_I_light_energy,Qdot_I_electricity_energy,Qdot_H_energy,Qdot_C_energy
  Bus Creator1 : BusCreator  Inputs=13
  Bus Selector1 : BusSelector  OutputSignals=z10.Qdot_T_opaque,z10.Qdot_T_ground,z10.Qdot_T_neighbour,z10.Qdot_T_window,z10.Qdot_V_mech,z10.Qdot_V_window,z10.Qdot_V_infiltration,z10.Qdot_S,z10.Qdot_I_person,z10.Qdot_I_light,z10.Qdot_I_electricity,z10.Qdot_H,z10.Qdot_C
  Constant{,1..12} (13 alike) : Constant  Value=0
  Subsystem : Subsystem
  Subsystem1 : Subsystem
  Subsystem10 : Subsystem
  Subsystem11 : Subsystem
  Subsystem12 : Subsystem
  Subsystem2 : Subsystem
  Subsystem3 : Subsystem
  Subsystem4 : Subsystem
  Subsystem5 : Subsystem
  Subsystem6 : Subsystem
  Subsystem7 : Subsystem
  Subsystem8 : Subsystem
  Subsystem9 : Subsystem
  BDBenergy : Outport
  wires:
  Subsystem1/1(Out1) -> Bus Assignment/3
  Subsystem2/1(Out1) -> Bus Assignment/4
  Subsystem3/1(Out1) -> Bus Assignment/5
  Subsystem4/1(Out1) -> Bus Assignment/6
  Subsystem5/1(Out1) -> Bus Assignment/7
  Subsystem6/1(Out1) -> Bus Assignment/8
  Subsystem7/1(Out1) -> Bus Assignment/9
  Subsystem8/1(Out1) -> Bus Assignment/10
  Subsystem9/1(Out1) -> Bus Assignment/11
  Subsystem10/1(Out1) -> Bus Assignment/12
  Subsystem11/1(Out1) -> Bus Assignment/13
  Subsystem12/1(Out1) -> Bus Assignment/14
  Subsystem/1(Out1) -> Bus Assignment/2
  Bus Creator1/1 -> Bus Assignment/1
  Bus Assignment/1 -> BDBenergy/1
  Bus Selector1/5 -> Subsystem4/1(In1)  "<Qdot_V_mech>"
  Bus Selector1/6 -> Subsystem5/1(In1)  "<Qdot_V_window>"
  Bus Selector1/7 -> Subsystem6/1(In1)  "<Qdot_V_infiltration>"
  Bus Selector1/8 -> Subsystem7/1(In1)  "<Qdot_S>"
  Bus Selector1/13 -> Subsystem12/1(In1)  "<Qdot_C>"
  Bus Selector1/12 -> Subsystem11/1(In1)  "<Qdot_H>"
  Bus Selector1/11 -> Subsystem10/1(In1)  "<Qdot_I_electricity>"
  Bus Selector1/10 -> Subsystem9/1(In1)  "<Qdot_I_light>"
  Bus Selector1/9 -> Subsystem8/1(In1)  "<Qdot_I_person>"
  Bus Selector1/2 -> Subsystem1/1(In1)  "<Qdot_T_ground>"
  Bus Selector1/3 -> Subsystem2/1(In1)  "<Qdot_T_neighbour>"
  Bus Selector1/4 -> Subsystem3/1(In1)  "<Qdot_T_window>"
  Bus Selector1/1 -> Subsystem/1(In1)  "<Qdot_T_opaque>"
  Constant5/1 -> Bus Creator1/6  "Qdot_V_window_energy"
  BDB/1 -> Bus Selector1/1
  Constant6/1 -> Bus Creator1/7  "Qdot_V_infiltration_energy"
  Constant7/1 -> Bus Creator1/9  "Qdot_I_person_energy"
  Constant8/1 -> Bus Creator1/8  "Qdot_S_energy"
  Constant/1 -> Bus Creator1/1  "Qdot_T_opaque_energy"
  Constant10/1 -> Bus Creator1/11  "Qdot_I_electricity_energy"
  Constant11/1 -> Bus Creator1/12  "Qdot_H_energy"
  Constant3/1 -> Bus Creator1/4  "Qdot_T_window_energy"
  Constant1/1 -> Bus Creator1/2  "Qdot_T_ground_energy"
  Constant9/1 -> Bus Creator1/10  "Qdot_I_light_energy"
  Constant4/1 -> Bus Creator1/5  "Qdot_V_mech_energy"
  Constant2/1 -> Bus Creator1/3  "Qdot_T_neighbour_energy"
  Constant12/1 -> Bus Creator1/13  "Qdot_C_energy"
